simulink model "a3"  (R2015b)
settings: Solver=VariableStepAuto  StartTime=0.0  StopTime=10.0  RelTol=1e-3
settings Model: Creator=Admin  LastModifiedBy=Admin

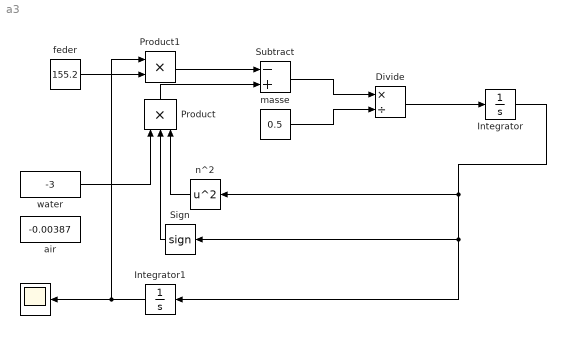
== system a3 ==
  " " : Scope
  Divide : Product  Inputs=*/
  Integrator : Integrator
  Integrator1 : Integrator  InitialCondition=1
  Product : Product  Inputs=3
  Product1 : Product
  Sign : Signum
  Subtract : Sum  Inputs=-+
  air : Constant  Value=-0.00387
  feder : Constant  Value=155.2
  masse : Constant  Value=0.5
  n^2 : Math  Operator=square  SaturateOnIntegerOverflow=on
  water : Constant  Value=-3
  wires:
  Integrator/1 -> Integrator1/1, Sign/1, n^2/1
  Integrator1/1 -> " "/1, Product1/1
  feder/1 -> Product1/2
  Product/1 -> Subtract/2
  Product1/1 -> Subtract/1
  Subtract/1 -> Divide/1
  masse/1 -> Divide/2
  Divide/1 -> Integrator/1
  n^2/1 -> Product/3
  Sign/1 -> Product/2
  water/1 -> Product/1
